simulink model "Model_1"  (R2024a)
settings: Solver=VariableStepAuto  StartTime=0.0  StopTime=10.0  RelTol=1e-3
settings Model: Creator=10232  LastModifiedBy=10232

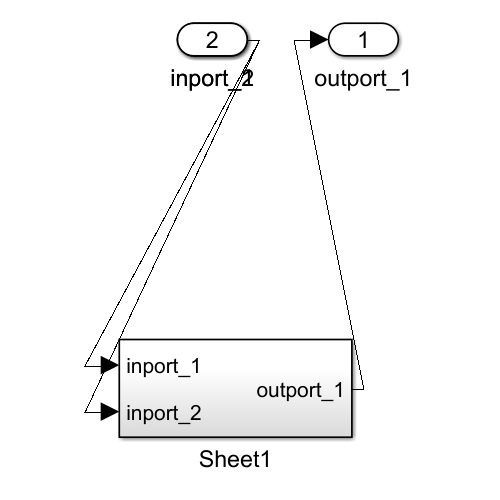
[thumbnail: Simulink's stored preview of the top-level diagram]
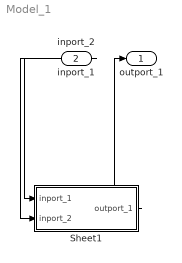
== system Model_1 ==
  inport_1 : Inport  OutDataTypeStr=single
  inport_2 : Inport  Port=2  OutDataTypeStr=int16
  Sheet1 : Subsystem
  outport_1 : Outport  OutDataTypeStr=uint16
  wires:
  inport_1/1 -> Sheet1/1(inport_1)
  Sheet1/1(outport_1) -> outport_1/1
  inport_2/1 -> Sheet1/2(inport_2)

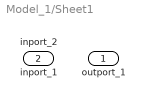
== system Model_1/Sheet1 ==
  inport_1 : Inport  OutDataTypeStr=single
  inport_2 : Inport  Port=2  OutDataTypeStr=int16
  outport_1 : Outport  OutDataTypeStr=uint16
